simulink model "test1"  (R2016a)
settings: Solver=FixedStepAuto  SolverMode=SingleTasking  StartTime=0.0  StopTime=10.0  RelTol=1e-3
PreLoadFcn:
  | waijung.modelPreload; % Required for working with Waijung Blockset. Do not remove.
libraries: powerlib x14, powerlib_meascontrol x1, simulink x1
CloseFcn:
  | waijung.modelClose; % Required for working with Waijung Blockset. Do not remove.
settings Model: Creator=Dang Khoa  LastModifiedBy=Dang Khoa
settings OptimizationCC: DefaultParameterBehavior=Inlined  OptimizeModelRefInitCode=on  LifeSpan=1
settings HardwareCC: ProdBitPerPointer=32  ProdLargestAtomicFloat=None  ProdIntDivRoundTo=Undefined  ProdWordSize=32  ProdHWDeviceType=ARM Compatible->Cortex - M4  TargetEndianess=LittleEndian  TargetHWDeviceType=ARM Compatible->Cortex - M4
settings RTWCC: SystemTargetFile=stm32f4.tlc  GenerateMakefile=off  TemplateMakefile=ert_default_tmf  Description=STM32F4 Target  GenerateReport=on  IncludeHyperlinkInReport=on  LaunchReport=on  GenerateTraceInfo=on  GenerateTraceReport=on  GenerateTraceReportSl=on  GenerateTraceReportSf=on  GenerateTraceReportEml=on
settings CodeAppCC: ForceParamTrailComments=on  IgnoreCustomStorageClasses=off  OperatorAnnotations=on  SimulinkDataObjDesc=on  SFDataObjDesc=on  MATLABFcnDesc=on  InsertBlockDesc=on  MATLABSourceComments=on
settings STFCustomTargetCC: ModelReferenceCompliant=off  CombineOutputUpdateFcns=on  ERTCustomFileBanners=on  SupportContinuousTime=off  SupportNonInlinedSFcns=off  MATLABClassNameForMDSCustomization=Simulink.SoftwareTarget.ERTCustomization  GRTInterface=off  SystemTargetFile=stm32f4.tlc
settings ERTTargetCC: ModelReferenceCompliant=off  ParMdlRefBuildCompliant=off  CompOptLevelCompliant=off  ConcurrentExecutionCompliant=off  ERTFirstTimeCompliant=off  ModelStepFunctionPrototypeControlCompliant=off  CPPClassGenCompliant=off  UseToolchainInfoCompliant=off  InlinedParameterPlacement=NonHierarchical  ERTSrcFileBannerTemplate=stm32f4_code_template.cgt  ERTHdrFileBannerTemplate=stm32f4_code_template.cgt  ERTDataSrcFileTemplate=stm32f4_code_template.cgt  ERTDataHdrFileTemplate=stm32f4_code_template.cgt  ERTCustomFileTemplate=stm32f4_file_process.tlc

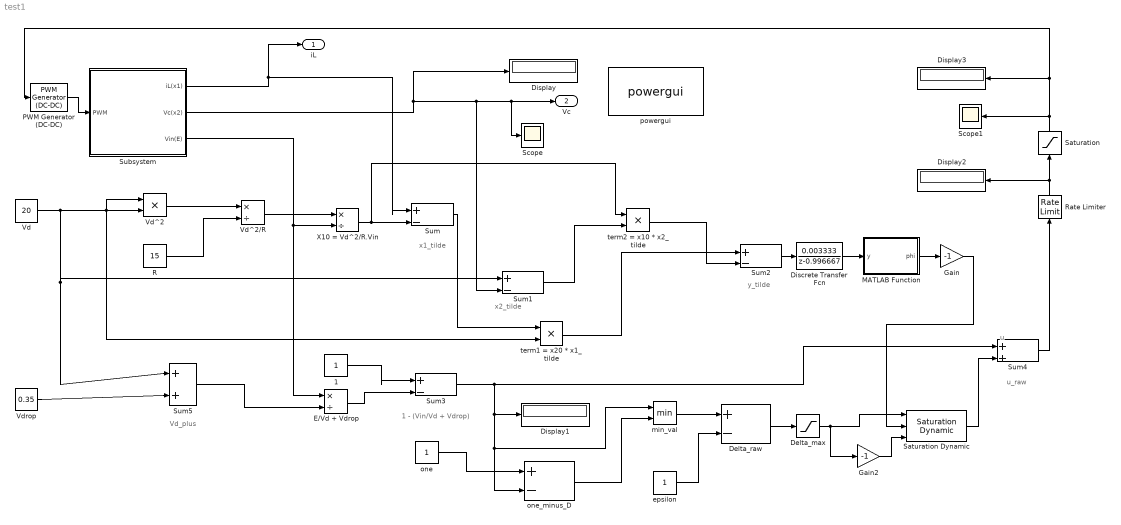
== system test1 ==
  note: Vd_plus
  note: u_raw
  note: u
  note: 1 - (Vin/Vd + Vdrop)
  note: x1_tilde
  note: x2_tilde
  note: y_tilde
  "1 " : Constant
  Delta_max : Saturate  UpperLimit=inf  LowerLimit=0
  Delta_raw : Sum  Inputs=+-
  Discrete Transfer Fcn : DiscreteTransferFcn  Numerator=[0.003333]  Denominator=[1 -0.996667]  SampleTime=5e-6
  Display{,1..3} (4 alike) : Display
  E/Vd + Vdrop : Product  Inputs=*/
  Gain : Gain  Gain=-1
  Gain2 : Gain  Gain=-1
  MATLAB Function : MATLAB Function  TreatAsAtomicUnit=on
  PWM Generator (DC-DC) : powerlib_meascontrol/Pulse & Signal Generators/PWM Generator (DC-DC)  Fsw=20000  Ts=5e-6
  R : Constant  Value=15
  Rate Limiter : RateLimiter  RisingSlewLimit=0.5  FallingSlewLimit=-0.5  SampleTimeMode=inherited
  Saturation : Saturate  UpperLimit=1  LowerLimit=0
  Saturation Dynamic : simulink/Discontinuities/Saturation Dynamic  OutMin=[]  OutMax=[]  OutDataTypeStr=Inherit: Same as second input  OutDataType=fixdt(1, 16)  OutScaling=2^-10  DoSatur=off
  Scope : Scope
  Scope1 : Scope
  Subsystem : Subsystem
  Sum{,1..3} (4 alike) : Sum  Inputs=|+-
  Sum4 : Sum  Inputs=|++
  Sum5 : Sum  Inputs=|++
  Vd : Constant  Value=20
  Vd^2 : Product
  Vd^2/R : Product  Inputs=*/
  Vdrop : Constant  Value=0.35
  X10 = Vd^2/R.Vin : Product  Inputs=*/
  epsilon : Constant
  min_val : MinMax  Inputs=2
  one : Constant
  one_minus_D : Sum  Inputs=+-
  powergui : powerlib/powergui  Priority=1  SimulationMode=Discrete  SolverType=Tustin/Backward Euler (TBE)  SampleTime=5e-6  frequency=60  SPID=off  DisableSnubberDevices=off  DisableRonSwitches=off  DisableVfSwitches=off  SwTol=0  DisplayEquations=off  Interpol=off  ExternalGateDelay=off  methode=off  Ts=10  FunctionMessages=off  echomessages=off  HookPort=off  EnableUseOfTLC=off  x0status=blocks  frequencyindice=0  Pbase=100e6  ErrMax=1e-4  Iterations=50  UnitsV=kV  UnitsW=MW  buscounter=0  RestoreLinks=warning  ResistiveCurrentMeasurement=off  Frange=[0:2:500]  Ylog=off  Xlog=on  ShowGrid=off  save=off  variable=ZData  structure=0  ZoomFFT=off  StartTime=0.0  cycles=1  DisplayStyle=1  fundamental=60  FreqAxis=off  MaxFrequency=1000  frequencyindicesteady=1  RmsSteady=1  display=off
  term1 = x20 * x1_tilde : Product
  term2 = x10 * x2_tilde : Product
  iL : Outport
  Vc : Outport  Port=2
  wires:
  PWM Generator (DC-DC)/1 -> Subsystem/1(PWM)
  Subsystem/1(iL(x1)) -> iL/1, Sum/1
  Vd/1 -> Sum1/1, Sum5/1, term1 = x20 * x1_tilde/2, Vd^2/1, Vd^2/2
  Vd^2/1 -> Vd^2/R/1
  R/1 -> Vd^2/R/2
  Vd^2/R/1 -> X10 = Vd^2/R.Vin/1
  Subsystem/3(Vin(E)) -> E/Vd + Vdrop/1, X10 = Vd^2/R.Vin/2
  X10 = Vd^2/R.Vin/1 -> term2 = x10 * x2_tilde/1, Sum/2
  Subsystem/2(Vc(x2)) -> Display/1, Sum1/2, Scope/1, Vc/1
  Sum/1 -> term1 = x20 * x1_tilde/1
  Sum1/1 -> term2 = x10 * x2_tilde/2
  term1 = x20 * x1_tilde/1 -> Sum2/1
  term2 = x10 * x2_tilde/1 -> Sum2/2
  MATLAB Function/1(phi) -> Gain/1
  "1 "/1 -> Sum3/1
  E/Vd + Vdrop/1 -> Sum3/2
  Sum3/1 -> Sum4/1, min_val/1, one_minus_D/2, Display1/1
  one/1 -> one_minus_D/1
  one_minus_D/1 -> min_val/2
  min_val/1 -> Delta_raw/1
  epsilon/1 -> Delta_raw/2
  Delta_raw/1 -> Delta_max/1
  Delta_max/1 -> Gain2/1, Saturation Dynamic/1
  Gain2/1 -> Saturation Dynamic/3
  Saturation Dynamic/1 -> Sum4/2
  Gain/1 -> Saturation Dynamic/2
  Sum2/1 -> Discrete Transfer Fcn/1
  Discrete Transfer Fcn/1 -> MATLAB Function/1(y)
  Vdrop/1 -> Sum5/2
  Sum5/1 -> E/Vd + Vdrop/2
  Sum4/1 -> Rate Limiter/1
  Rate Limiter/1 -> Saturation/1, Display2/1
  Saturation/1 -> Display3/1, PWM Generator (DC-DC)/1, Scope1/1

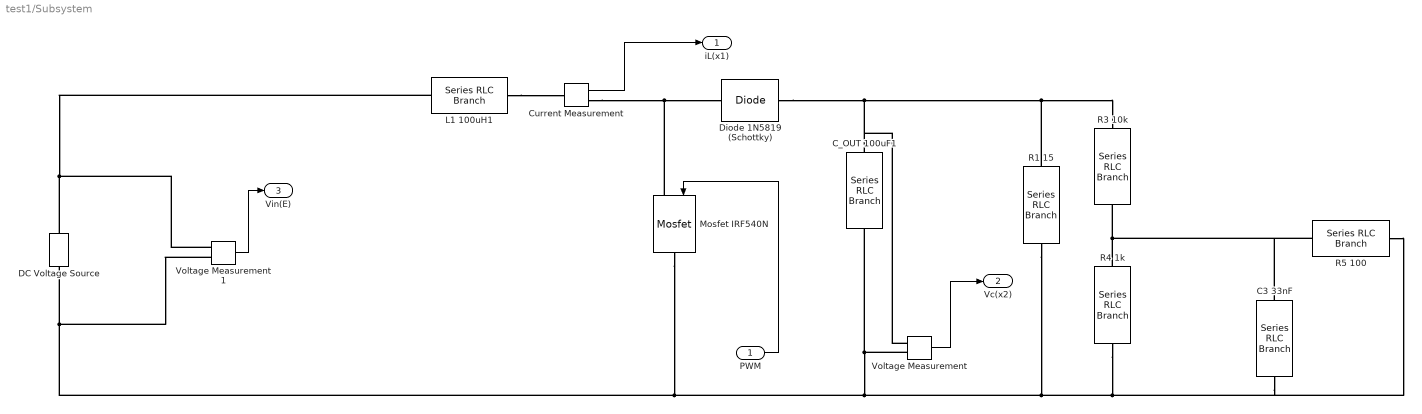
== system test1/Subsystem ==
  PWM : Inport
  C3 33nF : powerlib/Elements/Series RLC Branch  LConnTagsString=__new0  RConnTagsString=__new0  BranchType=C  Resistance=1  Inductance=1e-3  SetiL0=off  InitialCurrent=0  Capacitance=33e-9  Setx0=off  InitialVoltage=0  Measurements=None
  C_OUT 100uF1 : powerlib/Elements/Series RLC Branch  LConnTagsString=__new0  RConnTagsString=__new0  BranchType=C  Resistance=1  Inductance=1e-3  SetiL0=off  InitialCurrent=0  Capacitance=470e-6  Setx0=off  InitialVoltage=0  Measurements=None
  Current Measurement : powerlib/Measurements/Current Measurement  PhasorSimulation=off  OutputType=Complex  PSBequivalent=0
  DC Voltage Source : powerlib/Electrical Sources/DC Voltage Source  Amplitude=15  Measurements=None
  Diode 1N5819 (Schottky) : powerlib/Power Electronics/Diode  Ron=0.05  Lon=0  Vf=0.45  IC=0  UseSnubber=off  Rs=500  Cs=250e-12  Measurements=off
  L1 100uH1 : powerlib/Elements/Series RLC Branch  LConnTagsString=__new0  RConnTagsString=__new0  BranchType=L  Resistance=1  Inductance=100e-6  SetiL0=off  InitialCurrent=0  Capacitance=1e-6  Setx0=off  InitialVoltage=0  Measurements=None
  Mosfet IRF540N : powerlib/Power Electronics/Mosfet  Ron=0.01  Lon=0  Rd=0.01  Vfd=0  IC=0  Rs=inf  Cs=inf  Measurements=off
  R1 15 : powerlib/Elements/Series RLC Branch  LConnTagsString=__new0  RConnTagsString=__new0  BranchType=R  Resistance=10  Inductance=1e-3  SetiL0=off  InitialCurrent=0  Capacitance=1e-6  Setx0=off  InitialVoltage=0  Measurements=None
  R3 10k : powerlib/Elements/Series RLC Branch  LConnTagsString=__new0  RConnTagsString=__new0  BranchType=R  Resistance=100000  Inductance=1e-3  SetiL0=off  InitialCurrent=0  Capacitance=1e-6  Setx0=off  InitialVoltage=0  Measurements=None
  R4 1k : powerlib/Elements/Series RLC Branch  LConnTagsString=__new0  RConnTagsString=__new0  BranchType=R  Resistance=10000  Inductance=1e-3  SetiL0=off  InitialCurrent=0  Capacitance=1e-6  Setx0=off  InitialVoltage=0  Measurements=None
  R5 100 : powerlib/Elements/Series RLC Branch  LConnTagsString=__new0  RConnTagsString=__new0  BranchType=R  Resistance=100  Inductance=1e-3  SetiL0=off  InitialCurrent=0  Capacitance=1e-6  Setx0=off  InitialVoltage=0  Measurements=None
  Voltage Measurement : powerlib/Measurements/Voltage Measurement  PhasorSimulation=off  OutputType=Complex  PSBequivalent=0
  Voltage Measurement1 : powerlib/Measurements/Voltage Measurement  PhasorSimulation=off  OutputType=Complex  PSBequivalent=0
  iL(x1) : Outport
  Vc(x2) : Outport  Port=2
  Vin(E) : Outport  Port=3
  wires:
  Voltage Measurement/1 -> Vc(x2)/1
  Voltage Measurement1/1 -> Vin(E)/1
  Current Measurement/1 -> iL(x1)/1
  PWM/1 -> Mosfet IRF540N/1
  connections:
  R4 1k/LConn1 -- C3 33nF/LConn1 -- R5 100/LConn1 -- R3 10k/RConn1
  Voltage Measurement/LConn2 -- C_OUT 100uF1/RConn1 -- R4 1k/RConn1 -- C3 33nF/RConn1 -- R5 100/RConn1 -- R1 15/RConn1 -- Mosfet IRF540N/RConn1 -- Voltage Measurement1/LConn2 -- DC Voltage Source/LConn1
  Mosfet IRF540N/LConn1 -- Diode 1N5819 (Schottky)/LConn1 -- Current Measurement/RConn1
  Diode 1N5819 (Schottky)/RConn1 -- C_OUT 100uF1/LConn1 -- Voltage Measurement/LConn1 -- R1 15/LConn1 -- R3 10k/LConn1
  DC Voltage Source/RConn1 -- L1 100uH1/LConn1 -- Voltage Measurement1/LConn1
  L1 100uH1/RConn1 -- Current Measurement/LConn1

== matlab function test1/MATLAB Function ==
  data: y input; phi output
function phi = PBCphi(y)
a1 = 1; 
a2 = 0.5; 
a3 = 0.02;   % đúng PL2, bạn giữ/tune được
phi = a1*y + a2*y^3 + a3*y^5;
end
